simulink model "untitled1"  (R2020b)
settings: Solver=ode4  StartTime=0.0  StopTime=10.0  FixedStep=0.05  RelTol=1e-3
values from neighbouring files (symbols this model uses):
  DES_POS = [pi/2,0]    [Alternative_Init.m]    (also in init.m = [0,0,0,0])
  INITIAL_CONDITIONS = [0,0,0,0]    [Alternative_Init.m]    (also in init.m = [pi/3,pi/2,0,0]; lqr_init.m = [pi + pi/12, -pi/12, 0, 0])
  KD_GAIN = [2,0;0,9]    [Alternative_Init.m]    (also in init.m = [9,0;0,9])
  KP_GAIN = [10,0;0,10]    [Alternative_Init.m]    (also in init.m = [80,0;0,25])
  PARAM = [m1,m2,I1,lc1,l2,lc2,I1,I2]    [Alternative_Init.m]    (also in init.m)
settings Model: Creator=gianl  LastModifiedBy=gianl
settings DataIOCC: ReturnWorkspaceOutputs=off

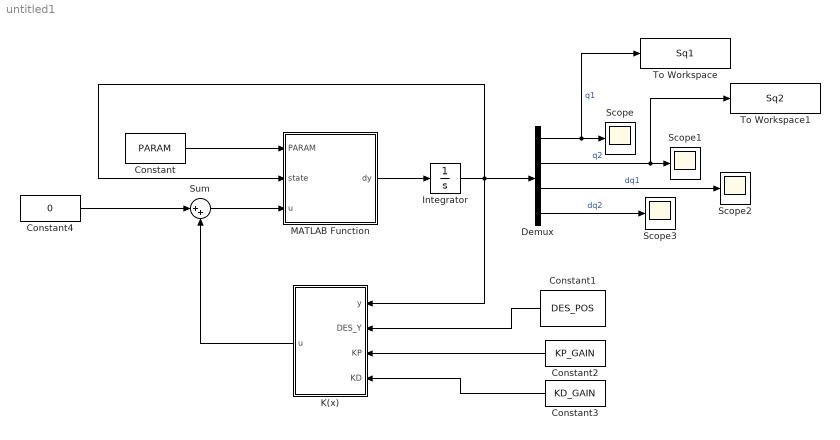
== system untitled1 ==
  Constant : Constant  Value=PARAM
  Constant1 : Constant  Value=DES_POS
  Constant2 : Constant  Value=KP_GAIN
  Constant3 : Constant  Value=KD_GAIN
  Constant4 : Constant  Value=0
  Demux : Demux
  Integrator : Integrator  InitialCondition=INITIAL_CONDITIONS
  K(x) : MATLAB Function  TreatAsAtomicUnit=on
  MATLAB Function : MATLAB Function  TreatAsAtomicUnit=on
  Scope{,1..3} (4 alike) : Scope
  Sum : Sum  Inputs=|++
  To Workspace : ToWorkspace  VariableName=Sq1  SaveFormat=Timeseries  SampleTime=-1
  To Workspace1 : ToWorkspace  VariableName=Sq2  SaveFormat=Timeseries  SampleTime=-1
  wires:
  Constant/1 -> MATLAB Function/1(PARAM)
  MATLAB Function/1(dy) -> Integrator/1
  Integrator/1 -> MATLAB Function/2(state), Demux/1, K(x)/1(y)
  K(x)/1(u) -> Sum/2
  Constant2/1 -> K(x)/3(KP)
  Constant1/1 -> K(x)/2(DES_Y)
  Demux/1 -> To Workspace/1, Scope/1  "q1"
  Demux/2 -> To Workspace1/1, Scope1/1  "q2"
  Demux/3 -> Scope2/1  "dq1"
  Demux/4 -> Scope3/1  "dq2"
  Constant3/1 -> K(x)/4(KD)
  Sum/1 -> MATLAB Function/3(u)
  Constant4/1 -> Sum/1

== matlab function untitled1/K(x) ==
  data: y input; DES_Y input; u output; KP input size=[2,2]; KD input size=[2,2]
function u = controller(y,DES_Y,KP,KD)
  
    posdes = [DES_Y(1),DES_Y(2)]';
    pos = [y(1),y(2)]';
    dpos = [y(3),y(4)]';
    u = KP*(posdes-pos)-KD*(dpos);
    %u=[u(1);0];
end

== matlab function untitled1/MATLAB Function ==
  data: PARAM input; state input; u input size=2; dy output size=4
function dy = nonlinearSys(PARAM,state,u)
m1 = PARAM(1);              % giunto 1 mass
m2 = PARAM(2);              % giunto 2 mass
l1 = PARAM(3);          % lunghezza primo giunto
lc1 = PARAM(4);          % centro di massa giunto 1
l2 = PARAM(5);
lc2 = PARAM(6);
I1 = PARAM(7);
I2 = PARAM(8);
g= 9.81;

q1 = state(1);
q2 = state(2);
dq1 = state(3);
dq2= state(4);

a1 = I1+ I2+ m1*lc1^2+m2*(l1^2+lc2^2);
a2 = m2*l1*lc2^2;
a3 = I2 + m2*lc2^2;
a4 = g*(m1*lc1+m2*l1);
a5 = g*m2*lc2;

M = [a1+2*a2*cos(q2), a3+a2*cos(q2);
     a3+a2*cos(q2), a3];
 
c = [-a2*dq2*(dq2+2*dq1)*sin(q2);
    a2*dq1^2*sin(q2)];
e = [ a4*sin(q1) + a5*sin(q1+q2);
    a5*sin(q1+q2)];
n = c+e;

f = [dq1;
    dq2;
    -inv(M)*n;
   ];

g =[0,0;
    0,0;
    inv(M);
    ];
dy =f+g*u;
